simulink subsystem "D1_Kerek"  (R2024b)
settings: Solver=VariableStepAuto  StartTime=0.0  StopTime=10.0  RelTol=1e-3
undefined symbols (not defined in the file or in its folder): b, C
settings Model: Creator=Asus  LastModifiedBy=Asus

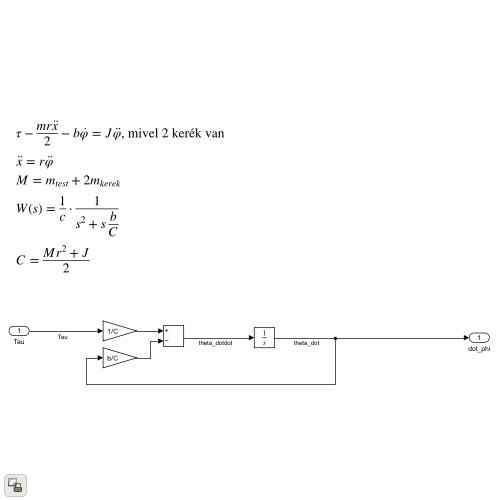
[thumbnail: Simulink's stored preview of the top-level diagram]
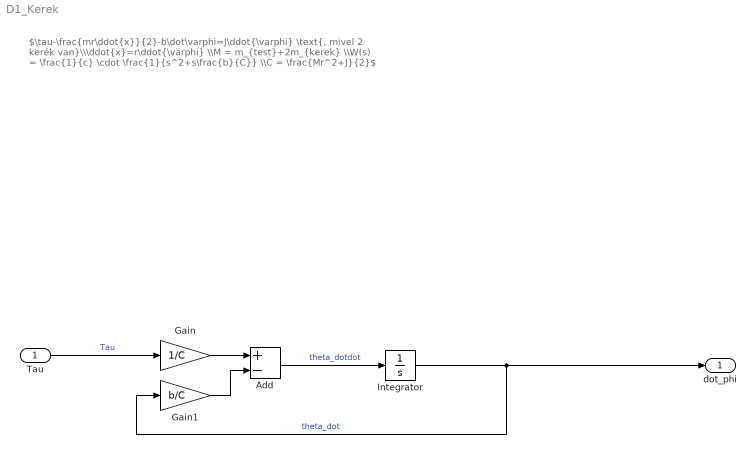
== system D1_Kerek ==
  note: $\tau-\frac{mr\ddot{x}}{2}-b\dot\varphi=J\ddot{\varphi} \text{, mivel 2 kerék van}\\\ddot{x}=r\ddot{\varphi} \\M = m_{test}+2m_{kerek} \\W(s) = \frac{1}{c} \cdot \frac{1}{s^2+s\frac{b}{C}} \\C = \frac{Mr^2+J}{2}$
  Tau : Inport
  Add : Sum  Inputs=+-
  Gain : Gain  Gain=1/C
  Gain1 : Gain  Gain=b/C
  Integrator : Integrator
  dot_phi : Outport
  wires:
  Tau/1 -> Gain/1  "Tau"
  Add/1 -> Integrator/1  "theta_dotdot"
  Integrator/1 -> dot_phi/1, Gain1/1  "theta_dot"
  Gain/1 -> Add/1
  Gain1/1 -> Add/2
